simulink model "ScriptDemo"  (R2022b)
settings: configuration reference "TmVcThermal_Configuration_sub" (kept outside this file)
undefined symbols (not defined in the file or in its folder): aaaa, bbbb, cTmComprCtrl_D_u8HvacFlowTable_db, cTmComprCtrl_D_u8HvacFlowTable_sw, cTmComprCtrl_n_i16ChillCmpIMax, cTmComprCtrl_n_i16ChillCmpIMin, cTmComprCtrl_n_i16ChillCmpIMin666, cTmComprCtrl_n_i16ChillCmpPMax, cTmComprCtrl_n_i16ChillCmpPMin, cTmComprCtrl_n_i16CmpChillCoolRpmKiMax, cTmComprCtrl_n_i16CmpChillCoolRpmKiMin, cTmComprCtrl_n_i16CmpChillCoolRpmKpMax, cTmComprCtrl_n_i16CmpChillCoolRpmKpMin, cTmComprCtrl_n_i16CmpCoolRpmKiMax, cTmComprCtrl_n_i16CmpCoolRpmKiMin, cTmComprCtrl_n_i16CmpCoolRpmKpMax, cTmComprCtrl_n_i16CmpCoolRpmKpMin, cTmComprCtrl_n_i16SM4CmpHeatKiMax, cTmComprCtrl_n_i16SM4CmpHeatKiMin, cTmComprCtrl_n_i16SM4CmpHeatKpMax, cTmComprCtrl_n_i16SM4CmpHeatKpMin, cTmComprCtrl_n_i16SM5CmpHeatKiMax, cTmComprCtrl_n_i16SM5CmpHeatKiMin, cTmComprCtrl_n_i16SM5CmpHeatKpMax, cTmComprCtrl_n_i16SM5CmpHeatKpMin, cTmComprCtrl_n_i16SM6CmpHeatKiMax, cTmComprCtrl_n_i16SM6CmpHeatKiMin, cTmComprCtrl_n_i16SM6CmpHeatKpMax, cTmComprCtrl_n_i16SM6CmpHeatKpMin, cTmComprCtrl_n_u16CmpMaxSpdFanFltLimt, cTmComprCtrl_n_u16CmpMaxSpdLoSidePFltLimt, cTmComprCtrl_n_u16CmpMaxSpdSensorFltLimt, cTmComprCtrl_n_u16CompMinRpm, cTmComprCtrl_n_u16CompRpmIncThres, cTmComprCtrl_t_u16BattCooltFFPeriod, cTmComprCtrl_t_u16BattCooltPIPeriod, cTmComprCtrl_t_u16CmpCoolFFPeriod, cTmComprCtrl_t_u16CmpCoolPIPeriod, cTmComprCtrl_t_u16CoolCmpChillFFPeriod, cTmComprCtrl_t_u16CoolCmpChillPIPeriod, cTmComprCtrl_t_u16SM4CmpHeatFFPeriod, cTmComprCtrl_t_u16SM4CmpHeatPIPeriod, cTmComprCtrl_t_u16SM5CmpHeatFFPeriod, cTmComprCtrl_t_u16SM5CmpHeatPIPeriod, cTmComprCtrl_t_u16SM6CmpHeatFFPeriod, cTmComprCtrl_t_u16SM6CmpHeatPIPeriod, cTmComprCtrl_Te_EvapClearInteg, cTmComprCtrl_Te_i16HpReqTempSaturoffset, cTmComprCtrl_Te_i16SatLpReplaceDiff, cTmComprCtrl_Te_i16SM3BatDiffStartEvapDecOffset, cTmComprCtrl_Te_i16SM3EvapLo, cTmComprCtrl_Te_i16SM3TBatDiffEntEvapDecOffset, cTmComprCtrl_Te_i16SM3TBatDiffEntEvapDecOffsetQuit, cTmComprCtrl_Te_s32ErrCmpChillPIContinueCoolH, cTmComprCtrl_Te_s32ErrCmpChillPIContinueCoolL, cTmComprCtrl_Te_s32ErrCmpPIContinueChillH, cTmComprCtrl_Te_s32ErrCmpPIContinueChillL, cTmComprCtrl_Te_s32ErrCmpPIContinueCoolH, cTmComprCtrl_Te_s32ErrCmpPIContinueCoolL, cTmComprCtrl_Te_s32ErrCmpPIContinueHeatH ... (+398)
libraries: simulink x846, PCMULib x711, simulink_need_slupdate x4
(part 33 of 49)

== system ScriptDemo/Create/createMerge/After/SM2SM22/SM2_Kp/Rec ==
  md_u8Blw : Inport
  breakpoint1 : Inport  Port=2
  breakpoint2 : Inport  Port=3
  2-D Lookup Table5 : Lookup_n-D  BreakpointsForDimension1=FFBlw1_Y  BreakpointsForDimension2=FFBlw1_X  BreakpointsForDimension1DataTypeStr=Inherit: Inherit from 'Breakpoint data'  BreakpointsForDimension2DataTypeStr=Inherit: Inherit from 'Breakpoint data'  Table=FFBlw1  TableDataTypeStr=Inherit: Inherit from 'Table data'  ExtrapMethod=Clip  InternalRulePriority=Speed  OutDataTypeStr=Inherit: Inherit from 'Table data'  RndMeth=Simplest
      settings: InputPortMap=u0,u1
  2-D Lookup Table6 : Lookup_n-D  BreakpointsForDimension1=FFBlw3_Y  BreakpointsForDimension2=FFBlw3_X  BreakpointsForDimension1DataTypeStr=Inherit: Inherit from 'Breakpoint data'  BreakpointsForDimension2DataTypeStr=Inherit: Inherit from 'Breakpoint data'  Table=FFBlw3  TableDataTypeStr=Inherit: Inherit from 'Table data'  ExtrapMethod=Clip  InternalRulePriority=Speed  OutDataTypeStr=Inherit: Inherit from 'Table data'  RndMeth=Simplest
      settings: InputPortMap=u0,u1
  2-D Lookup Table7 : Lookup_n-D  BreakpointsForDimension1=FFBlw5_Y  BreakpointsForDimension2=FFBlw5_X  BreakpointsForDimension1DataTypeStr=Inherit: Inherit from 'Breakpoint data'  BreakpointsForDimension2DataTypeStr=Inherit: Inherit from 'Breakpoint data'  Table=FFBlw5  TableDataTypeStr=Inherit: Inherit from 'Table data'  ExtrapMethod=Clip  InternalRulePriority=Speed  OutDataTypeStr=Inherit: Inherit from 'Table data'  RndMeth=Simplest
      settings: InputPortMap=u0,u1
  2-D Lookup Table8 : Lookup_n-D  BreakpointsForDimension1=FFBlw7_Y  BreakpointsForDimension2=FFBlw7_X  BreakpointsForDimension1DataTypeStr=Inherit: Inherit from 'Breakpoint data'  BreakpointsForDimension2DataTypeStr=Inherit: Inherit from 'Breakpoint data'  Table=FFBlw7  TableDataTypeStr=Inherit: Inherit from 'Table data'  ExtrapMethod=Clip  InternalRulePriority=Speed  OutDataTypeStr=Inherit: Inherit from 'Table data'  RndMeth=Simplest
      settings: InputPortMap=u0,u1
  2-D Lookup Table9 : Lookup_n-D  BreakpointsForDimension1=FFBlw9_Y  BreakpointsForDimension2=FFBlw9_X  BreakpointsForDimension1DataTypeStr=Inherit: Inherit from 'Breakpoint data'  BreakpointsForDimension2DataTypeStr=Inherit: Inherit from 'Breakpoint data'  Table=FFBlw9  TableDataTypeStr=Inherit: Inherit from 'Table data'  ExtrapMethod=Clip  InternalRulePriority=Speed  OutDataTypeStr=Inherit: Inherit from 'Table data'  RndMeth=Simplest
      settings: InputPortMap=u0,u1
  Add{2..6} (5 alike) : Sum  Inputs=+-  OutDataTypeStr=int16
  Add7 : Sum  Inputs=+++++
  Constant{,1..4} (5 alike) : Constant  Value=0.1  OutDataTypeStr=single
  Constant5 : Constant  Value=10  OutDataTypeStr=int16
  Constant6 : Constant  Value=20  OutDataTypeStr=int16
  Constant7 : Constant  Value=30  OutDataTypeStr=int16
  Constant8 : Constant  Value=40  OutDataTypeStr=int16
  Constant9 : Constant  Value=50  OutDataTypeStr=int16
  Data Type Conversion : DataTypeConversion  OutDataTypeStr=uint16  SaturateOnIntegerOverflow=off  RndMeth=Floor
  Data Type Conversion1 : DataTypeConversion  OutDataTypeStr=int16  SaturateOnIntegerOverflow=off  RndMeth=Floor
  Product{,1..9} (10 alike) : Product  OutDataTypeStr=single
  Subsystem1 : Subsystem
  Subsystem2 : Subsystem
  Subsystem3 : Subsystem
  Subsystem4 : Subsystem
  Subsystem5 : Subsystem
  XCP : Subsystem
  Flow2Rpm : Outport
  wires:
  Subsystem1/1(Out1) -> Product/2
  Product2/1 -> Product7/2
  [breakpoint2] -> 2-D Lookup Table5/2
  Product4/1 -> Product9/2
  Product9/1 -> Add7/5
  [breakpoint1] -> 2-D Lookup Table7/1
  Constant9/1 -> Add6/1
  [breakpoint1] -> 2-D Lookup Table9/1
  [breakpoint1] -> 2-D Lookup Table5/1
  [breakpoint1] -> 2-D Lookup Table6/1
  Product5/1 -> Add7/1
  2-D Lookup Table7/1 -> Product2/1
  Data Type Conversion1/1 -> Add4/2, Add6/2, Add5/2, Add3/2, Add2/2
  [breakpoint2] -> 2-D Lookup Table8/2
  Product/1 -> Product5/2
  Subsystem5/1(Out1) -> Product4/2
  [breakpoint2] -> 2-D Lookup Table7/2
  Subsystem2/1(Out1) -> Product1/2
  Constant8/1 -> Add5/1
  Product8/1 -> Add7/4
  Constant7/1 -> Add4/1
  Add4/1 -> Subsystem3/1(In1)
  Subsystem3/1(Out1) -> Product2/2
  Subsystem4/1(Out1) -> Product3/2
  Product1/1 -> Product6/2
  Add2/1 -> Subsystem1/1(In1)
  [breakpoint1] -> 2-D Lookup Table8/1
  [breakpoint2] -> 2-D Lookup Table6/2
  2-D Lookup Table5/1 -> Product/1
  Constant5/1 -> Add2/1
  2-D Lookup Table8/1 -> Product3/1
  Constant6/1 -> Add3/1
  Add6/1 -> Subsystem5/1(In1)
  Add5/1 -> Subsystem4/1(In1)
  Product3/1 -> Product8/2
  [breakpoint2] -> 2-D Lookup Table9/2
  Add3/1 -> Subsystem2/1(In1)
  Add7/1 -> Data Type Conversion/1
  2-D Lookup Table6/1 -> Product1/1
  Product7/1 -> Add7/3
  2-D Lookup Table9/1 -> Product4/1
  Product6/1 -> Add7/2
  breakpoint1/1 -> [breakpoint1]
  breakpoint2/1 -> [breakpoint2]
  XCP/1(Out1) -> Data Type Conversion1/1
  Constant/1 -> Product5/1
  Constant1/1 -> Product6/1
  Constant2/1 -> Product7/1
  Constant3/1 -> Product8/1
  Constant4/1 -> Product9/1
  md_u8Blw/1 -> XCP/1(md_u8Blw)
  Data Type Conversion/1 -> Flow2Rpm/1

== system ScriptDemo/Create/createMerge/After/SM3SM23/ID26262_SM3FF/SM1FFEnable ==
  xTmComprCtrl_B_CompOnReqCompOn : Inport  OutDataTypeStr=boolean
  BevvFFPeriod : Subsystem  mask{CounterLim=cTmComprCtrl_t_u16BattCooltFFPeriod}
      mask DialogControl ParameterGroupVar Prompt: 参数
  Compare To Constant2 : simulink/Logic and Bit Operations/Compare To Constant  relop===  const=0  OutDataTypeStr=boolean
  Compare To Constant3 : simulink/Logic and Bit Operations/Compare To Constant  relop===  const=1  OutDataTypeStr=boolean
  Logical Operator3 : Logic  AllPortsSameDT=off  OutDataTypeStr=boolean
  Unit Delay : UnitDelay  SampleTime=-1  HasFrameUpgradeWarning=on
  SM1FFEnable_B_SM1FFEnable : Outport  OutDataTypeStr=boolean
  wires:
  Unit Delay/1 -> Compare To Constant2/1
  [xTmComprCtrl_B_CompOnReqCompOn] -> Compare To Constant3/1, Unit Delay/1
  Compare To Constant2/1 -> Logical Operator3/1
  Logical Operator3/1 -> BevvFFPeriod/1(Counter_Reset)
  BevvFFPeriod/1(Counter_Trig) -> SM1FFEnable_B_SM1FFEnable/1
  Compare To Constant3/1 -> Logical Operator3/2
  xTmComprCtrl_B_CompOnReqCompOn/1 -> [xTmComprCtrl_B_CompOnReqCompOn]

== system ScriptDemo/Create/createMerge/After/SM3SM23/ID26262_SM3FF/SM2FFEnable ==
  xTmComprCtrl_B_CompOnReqCompOn : Inport  OutDataTypeStr=boolean
  Compare To Constant2 : simulink/Logic and Bit Operations/Compare To Constant  relop===  const=0  OutDataTypeStr=boolean
  Compare To Constant3 : simulink/Logic and Bit Operations/Compare To Constant  relop===  const=1  OutDataTypeStr=boolean
  Logical Operator3 : Logic  AllPortsSameDT=off  OutDataTypeStr=boolean
  PeriodTrig : Subsystem  mask{CounterLim=cTmComprCtrl_t_u16CoolCmpChillFFPeriod}
      mask DialogControl ParameterGroupVar Prompt: 参数
  Unit Delay : UnitDelay  SampleTime=-1  HasFrameUpgradeWarning=on
  SM2FFEnable_B_SM2FFEnable : Outport  OutDataTypeStr=boolean
  wires:
  Unit Delay/1 -> Compare To Constant2/1
  [xTmComprCtrl_B_CompOnReqCompOn] -> Compare To Constant3/1, Unit Delay/1
  Compare To Constant2/1 -> Logical Operator3/1
  Logical Operator3/1 -> PeriodTrig/1(Counter_Reset)
  Compare To Constant3/1 -> Logical Operator3/2
  xTmComprCtrl_B_CompOnReqCompOn/1 -> [xTmComprCtrl_B_CompOnReqCompOn]
  PeriodTrig/1(Counter_Trig) -> SM2FFEnable_B_SM2FFEnable/1

== system ScriptDemo/Create/createMerge/After/SM3SM23/ID26262_SM3FF/SM3SM1FF ==
  sTmIn_D_u8DCChrgSt : Inport  OutDataTypeStr=uint8
  sTmSigProces_D_u8HvBattCoolgReq : Inport  Port=2  OutDataTypeStr=uint8
  sTmIn_D_u8HeatPump : Inport  Port=3  OutDataTypeStr=uint8
  Enable : EnablePort
  1-D Lookup Table1 : Lookup_n-D  NumberOfTableDimensions=1  BreakpointsForDimension1=tTmComprCtrl_fac_s32SM1FFTFactor_X  BreakpointsForDimension1DataTypeStr=Inherit: Inherit from 'Breakpoint data'  Table=tTmComprCtrl_fac_s32SM1FFTFactor  TableDataTypeStr=Inherit: Inherit from 'Table data'  ExtrapMethod=Clip  InternalRulePriority=Speed  OutDataTypeStr=Inherit: Inherit via back propagation  RndMeth=Simplest  InputSameDT=off
  2-D Lookup Table1 : Lookup_n-D  BreakpointsForDimension1=mTmComprCtrl_n_u16FFBattCooltRpmNorm_Y  BreakpointsForDimension2=mTmComprCtrl_n_u16FFBattCooltRpmNorm_X  BreakpointsForDimension1DataTypeStr=Inherit: Inherit from 'Breakpoint data'  BreakpointsForDimension2DataTypeStr=Inherit: Inherit from 'Breakpoint data'  Table=mTmComprCtrl_n_u16FFBattCooltRpmNorm  TableDataTypeStr=Inherit: Inherit from 'Table data'  ExtrapMethod=Clip  InternalRulePriority=Speed  OutDataTypeStr=Inherit: Inherit via back propagation  RndMeth=Simplest  InputSameDT=off
      settings: InputPortMap=u0,u1
  2-D Lookup Table2 : Lookup_n-D  BreakpointsForDimension1=mTmComprCtrl_n_u16FFBattCooltRpmNormNhp_Y  BreakpointsForDimension2=mTmComprCtrl_n_u16FFBattCooltRpmNormNhp_X  BreakpointsForDimension1DataTypeStr=Inherit: Inherit from 'Breakpoint data'  BreakpointsForDimension2DataTypeStr=Inherit: Inherit from 'Breakpoint data'  Table=mTmComprCtrl_n_u16FFBattCooltRpmNormNhp  TableDataTypeStr=Inherit: Inherit from 'Table data'  ExtrapMethod=Clip  InternalRulePriority=Speed  OutDataTypeStr=Inherit: Inherit via back propagation  RndMeth=Simplest  InputSameDT=off
      settings: InputPortMap=u0,u1
  2-D Lookup Table5 : Lookup_n-D  LookupTableObject=mTmComprCtrl_n_u16FFBattCooltRpmCharging  BreakpointsForDimension1=mTmComprCtrl_n_u16FFBattCooltRpmChargingNhp_Y  BreakpointsForDimension2=mTmComprCtrl_n_u16FFBattCooltRpmChargingNhp_X  BreakpointsForDimension1DataTypeStr=Inherit: Inherit from 'Breakpoint data'  BreakpointsForDimension2DataTypeStr=Inherit: Inherit from 'Breakpoint data'  Table=mTmComprCtrl_n_u16FFBattCooltRpmChargingNhp  TableDataTypeStr=Inherit: Inherit from 'Table data'  ExtrapMethod=Clip  InternalRulePriority=Speed  OutDataTypeStr=Inherit: Inherit via back propagation  RndMeth=Simplest  InputSameDT=off
      settings: InputPortMap=u0,u1
  2-D Lookup Table6 : Lookup_n-D  LookupTableObject=mTmComprCtrl_n_u16FFBattCooltRpmCharging  BreakpointsForDimension1=mTmComprCtrl_n_u16FFBattCooltRpmCharging_Y  BreakpointsForDimension2=mTmComprCtrl_n_u16FFBattCooltRpmCharging_X  BreakpointsForDimension1DataTypeStr=Inherit: Inherit from 'Breakpoint data'  BreakpointsForDimension2DataTypeStr=Inherit: Inherit from 'Breakpoint data'  Table=mTmComprCtrl_n_u16FFBattCooltRpmCharging  TableDataTypeStr=Inherit: Inherit from 'Table data'  ExtrapMethod=Clip  InternalRulePriority=Speed  OutDataTypeStr=Inherit: Inherit via back propagation  RndMeth=Simplest  InputSameDT=off
      settings: InputPortMap=u0,u1
  2-D Lookup Table7 : Lookup_n-D  LookupTableObject=mTmComprCtrl_n_u16FFBattCooltRpmCharging  BreakpointsForDimension1=mTmComprCtrl_n_u16FFBattCooltRpmSuperCharging_Y  BreakpointsForDimension2=mTmComprCtrl_n_u16FFBattCooltRpmSuperCharging_X  BreakpointsForDimension1DataTypeStr=Inherit: Inherit from 'Breakpoint data'  BreakpointsForDimension2DataTypeStr=Inherit: Inherit from 'Breakpoint data'  Table=mTmComprCtrl_n_u16FFBattCooltRpmSuperCharging  TableDataTypeStr=Inherit: Inherit from 'Table data'  ExtrapMethod=Clip  InternalRulePriority=Speed  OutDataTypeStr=Inherit: Inherit via back propagation  RndMeth=Simplest  InputSameDT=off
      settings: InputPortMap=u0,u1
  2-D Lookup Table8 : Lookup_n-D  LookupTableObject=mTmComprCtrl_n_u16FFBattCooltRpmCharging  BreakpointsForDimension1=mTmComprCtrl_n_u16FFBattCooltRpmSuperChargingNhp_Y  BreakpointsForDimension2=mTmComprCtrl_n_u16FFBattCooltRpmSuperChargingNhp_X  BreakpointsForDimension1DataTypeStr=Inherit: Inherit from 'Breakpoint data'  BreakpointsForDimension2DataTypeStr=Inherit: Inherit from 'Breakpoint data'  Table=mTmComprCtrl_n_u16FFBattCooltRpmSuperChargingNhp  TableDataTypeStr=Inherit: Inherit from 'Table data'  ExtrapMethod=Clip  InternalRulePriority=Speed  OutDataTypeStr=Inherit: Inherit via back propagation  RndMeth=Simplest  InputSameDT=off
      settings: InputPortMap=u0,u1
  Compare To Constant : simulink/Logic and Bit Operations/Compare To Constant  relop===  const=2  OutDataTypeStr=boolean
  Multiport Switch : MultiPortSwitch  DataPortOrder=Specify indices  DataPortIndices={2,12}  DataPortForDefault=Additional data port  DiagnosticForDefault=None  SaturateOnIntegerOverflow=off  InputSameDT=off
  Multiport Switch1 : MultiPortSwitch  DataPortOrder=Specify indices  DataPortIndices={2,12}  DataPortForDefault=Additional data port  DiagnosticForDefault=None  SaturateOnIntegerOverflow=off  InputSameDT=off
  Product1 : Product  OutDataTypeStr=uint16
  Switch : Switch  Criteria=u2 ~= 0  SaturateOnIntegerOverflow=off  InputSameDT=off
  SM1FF : Outport
  wires:
  ? -> [sTmIn_Te_s32HvBattCooltTReq]
  sTmIn_D_u8DCChrgSt/1 -> [sTmIn_D_u8DCChrgSt]
  sTmSigProces_D_u8HvBattCoolgReq/1 -> [sTmSigProces_D_u8HvBattCoolgReq]
  ? -> [sTmSigProces_Te_s32TAmb]
  Multiport Switch1/1 -> Switch/3
  Switch/1 -> Product1/1  "rTmComprCtrl_fac_s32SM3SM1FFRaw"
  2-D Lookup Table5/1 -> Multiport Switch1/3
  [sTmSigProces_D_u8HvBattCoolgReq] -> 2-D Lookup Table8/1, 2-D Lookup Table5/1, 2-D Lookup Table2/1
  [sTmIn_D_u8DCChrgSt] -> Multiport Switch1/1
  2-D Lookup Table8/1 -> Multiport Switch1/4
  2-D Lookup Table2/1 -> Multiport Switch1/2
  2-D Lookup Table1/1 -> Multiport Switch/2
  Compare To Constant/1 -> Switch/2
  [sTmIn_D_u8DCChrgSt] -> Multiport Switch/1
  2-D Lookup Table6/1 -> Multiport Switch/3
  [sTmIn_D_u8HeatPump] -> Compare To Constant/1
  2-D Lookup Table7/1 -> Multiport Switch/4
  Multiport Switch/1 -> Switch/1
  [sTmSigProces_Te_s32TAmb] -> 1-D Lookup Table1/1
  Product1/1 -> SM1FF/1  "SM1FF"
  [sTmSigProces_D_u8HvBattCoolgReq] -> 2-D Lookup Table7/1, 2-D Lookup Table6/1, 2-D Lookup Table1/1
  1-D Lookup Table1/1 -> Product1/2  "rTmComprCtrl_fac_s32SM3SM1FFTFactor"
  [sTmIn_Te_s32HvBattCooltTReq] -> 2-D Lookup Table7/2, 2-D Lookup Table6/2, 2-D Lookup Table1/2
  [sTmIn_Te_s32HvBattCooltTReq] -> 2-D Lookup Table8/2, 2-D Lookup Table5/2, 2-D Lookup Table2/2
  sTmIn_D_u8HeatPump/1 -> [sTmIn_D_u8HeatPump]

== system ScriptDemo/Create/createMerge/After/SM3SM23/ID26262_SM3FF/SM3SM2FF ==
  note: FF
  sTmSigProces_Te_s32EvapFanReqRamp : Inport  OutDataTypeStr=single
  sTmIn_X_s32ClimtRcirc : Inport  Port=2  OutDataTypeStr=single
  sTmComprCtrl_D_u8HvacFlowLevel : Inport  Port=3  OutDataTypeStr=uint8
  sTmIn_D_u8HeatPump : Inport  Port=4  OutDataTypeStr=uint8
  Enable : EnablePort
  Compare To Constant : simulink/Logic and Bit Operations/Compare To Constant  relop===  const=2  OutDataTypeStr=boolean
  Demux : Demux  Outputs=2
  Flow2RpmOsa : Subsystem  mask{BlwHeatLevel_db=cTmComprCtrl_D_u8HvacFlowTable_db, BlwHeatLevel_sw=cTmComprCtrl_D_u8HvacFlowTable_sw, FFBlw1=mTmComprCtrl_n_u16FFCmpCoolRpm_OsaFlow1, FFBlw1_Y=mTmComprCtrl_n_u16FFCmpCoolRpm_OsaFlow1_Y, FFBlw1_X=mTmComprCtrl_n_u16FFCmpCoolRpm_OsaFlow1_X, FFBlw3=mTmComprCtrl_n_u16FFCmpCoolRpm_OsaFlow3, FFBlw3_Y=mTmComprCtrl_n_u16FFCmpCoolRpm_OsaFlow3_Y, FFBlw3_X=mTmComprCtrl_n_u16FFCmpCoolRpm_OsaFlow3_X, FFBlw5=mTmComprCtrl_n_u16FFCmpCoolRpm_OsaFlow5, FFBlw5_Y=mTmComprCtrl_n_u16FFCmpCoolRpm_OsaFlow5_Y, FFBlw5_X=mTmComprCtrl_n_u16FFCmpCoolRpm_OsaFlow5_X, FFBlw7=mTmComprCtrl_n_u16FFCmpCoolRpm_OsaFlow7, FFBlw7_Y=mTmComprCtrl_n_u16FFCmpCoolRpm_OsaFlow7_Y, FFBlw7_X=mTmComprCtrl_n_u16FFCmpCoolRpm_OsaFlow7_X, FFBlw9=mTmComprCtrl_n_u16FFCmpCoolRpm_OsaFlow9, FFBlw9_Y=mTmComprCtrl_n_u16FFCmpCoolRpm_OsaFlow9_Y, FFBlw9_X=mTmComprCtrl_n_u16FFCmpCoolRpm_OsaFlow9_X}
      mask DialogControl ParameterGroupVar Prompt: 参数
  Flow2RpmOsa1 : Subsystem  mask{BlwHeatLevel_db=cTmComprCtrl_D_u8HvacFlowTable_db, BlwHeatLevel_sw=cTmComprCtrl_D_u8HvacFlowTable_sw, FFBlw1=mTmComprCtrl_n_u16FFCmpCoolRpmNhpOsaFlow1, FFBlw1_Y=mTmComprCtrl_n_u16FFCmpCoolRpmNhpOsaFlow1_Y, FFBlw1_X=mTmComprCtrl_n_u16FFCmpCoolRpmNhpOsaFlow1_X, FFBlw3=mTmComprCtrl_n_u16FFCmpCoolRpmNhpOsaFlow3, FFBlw3_Y=mTmComprCtrl_n_u16FFCmpCoolRpmNhpOsaFlow3_Y, FFBlw3_X=mTmComprCtrl_n_u16FFCmpCoolRpmNhpOsaFlow3_X, FFBlw5=mTmComprCtrl_n_u16FFCmpCoolRpmNhpOsaFlow5, FFBlw5_Y=mTmComprCtrl_n_u16FFCmpCoolRpmNhpOsaFlow5_Y, FFBlw5_X=mTmComprCtrl_n_u16FFCmpCoolRpmNhpOsaFlow5_X, FFBlw7=mTmComprCtrl_n_u16FFCmpCoolRpmNhpOsaFlow7, FFBlw7_Y=mTmComprCtrl_n_u16FFCmpCoolRpmNhpOsaFlow7_Y, FFBlw7_X=mTmComprCtrl_n_u16FFCmpCoolRpmNhpOsaFlow7_X, FFBlw9=mTmComprCtrl_n_u16FFCmpCoolRpmNhpOsaFlow9, FFBlw9_Y=mTmComprCtrl_n_u16FFCmpCoolRpmNhpOsaFlow9_Y, FFBlw9_X=mTmComprCtrl_n_u16FFCmpCoolRpmNhpOsaFlow9_X}
      mask DialogControl ParameterGroupVar Prompt: 参数
  Flow2RpmRec : Subsystem  mask{BlwHeatLevel_db=cTmComprCtrl_D_u8HvacFlowTable_db, BlwHeatLevel_sw=cTmComprCtrl_D_u8HvacFlowTable_sw, FFBlw1=mTmComprCtrl_n_u16FFCmpCoolRpm_RecFlow1, FFBlw1_Y=mTmComprCtrl_n_u16FFCmpCoolRpm_RecFlow1_Y, FFBlw1_X=mTmComprCtrl_n_u16FFCmpCoolRpm_RecFlow1_X, FFBlw3=mTmComprCtrl_n_u16FFCmpCoolRpm_RecFlow3, FFBlw3_Y=mTmComprCtrl_n_u16FFCmpCoolRpm_RecFlow3_Y, FFBlw3_X=mTmComprCtrl_n_u16FFCmpCoolRpm_RecFlow3_X, FFBlw5=mTmComprCtrl_n_u16FFCmpCoolRpm_RecFlow5, FFBlw5_Y=mTmComprCtrl_n_u16FFCmpCoolRpm_RecFlow5_Y, FFBlw5_X=mTmComprCtrl_n_u16FFCmpCoolRpm_RecFlow5_X, FFBlw7=mTmComprCtrl_n_u16FFCmpCoolRpm_RecFlow7, FFBlw7_Y=mTmComprCtrl_n_u16FFCmpCoolRpm_RecFlow7_Y, FFBlw7_X=mTmComprCtrl_n_u16FFCmpCoolRpm_RecFlow7_X, FFBlw9=mTmComprCtrl_n_u16FFCmpCoolRpm_RecFlow9, FFBlw9_Y=mTmComprCtrl_n_u16FFCmpCoolRpm_RecFlow9_Y, FFBlw9_X=mTmComprCtrl_n_u16FFCmpCoolRpm_RecFlow9_X}
      mask DialogControl ParameterGroupVar Prompt: 参数
  Flow2RpmRec1 : Subsystem  mask{BlwHeatLevel_db=cTmComprCtrl_D_u8HvacFlowTable_db, BlwHeatLevel_sw=cTmComprCtrl_D_u8HvacFlowTable_sw, FFBlw1=mTmComprCtrl_n_u16FFCmpCoolRpmNhpRecFlow1, FFBlw1_Y=mTmComprCtrl_n_u16FFCmpCoolRpmNhpRecFlow1_Y, FFBlw1_X=mTmComprCtrl_n_u16FFCmpCoolRpmNhpRecFlow1_X, FFBlw3=mTmComprCtrl_n_u16FFCmpCoolRpmNhpRecFlow3, FFBlw3_Y=mTmComprCtrl_n_u16FFCmpCoolRpmNhpRecFlow3_Y, FFBlw3_X=mTmComprCtrl_n_u16FFCmpCoolRpmNhpRecFlow3_X, FFBlw5=mTmComprCtrl_n_u16FFCmpCoolRpmNhpRecFlow5, FFBlw5_Y=mTmComprCtrl_n_u16FFCmpCoolRpmNhpRecFlow5_Y, FFBlw5_X=mTmComprCtrl_n_u16FFCmpCoolRpmNhpRecFlow5_X, FFBlw7=mTmComprCtrl_n_u16FFCmpCoolRpmNhpRecFlow7, FFBlw7_Y=mTmComprCtrl_n_u16FFCmpCoolRpmNhpRecFlow7_Y, FFBlw7_X=mTmComprCtrl_n_u16FFCmpCoolRpmNhpRecFlow7_X, FFBlw9=mTmComprCtrl_n_u16FFCmpCoolRpmNhpRecFlow9, FFBlw9_Y=mTmComprCtrl_n_u16FFCmpCoolRpmNhpRecFlow9_Y, FFBlw9_X=mTmComprCtrl_n_u16FFCmpCoolRpmNhpRecFlow9_X}
      mask DialogControl ParameterGroupVar Prompt: 参数
  Mux : Mux  Inputs=2
  Mux1 : Mux  Inputs=2
  Signal Conversion : SignalConversion  OverrideOpt=off
  Signal Conversion1 : SignalConversion  OverrideOpt=off
  Switch : Switch  Criteria=u2 ~= 0  SaturateOnIntegerOverflow=off  InputSameDT=off
  interpolation : PCMULib/Calculation/interpolation  SystemSampleTime=-1  VariantActivationTime=update diagram  Latency=0  AutoFrameSizeCalculation=off
      settings: SourceProductName=PCMULib
  SM2FF : Outport  OutDataTypeStr=uint16
  wires:
  [sTmIn_X_s32ClimtRcirc] -> interpolation/1
  interpolation/1 -> SM2FF/1
  sTmSigProces_Te_s32EvapFanReqRamp/1 -> [sTmSigProces_Te_s32EvapFanReqRamp]
  ? -> [sTmSigProces_Te_s32TAmb]
  sTmIn_X_s32ClimtRcirc/1 -> [sTmIn_X_s32ClimtRcirc]
  sTmComprCtrl_D_u8HvacFlowLevel/1 -> [sTmComprCtrl_D_u8HvacFlowLevel]
  [sTmComprCtrl_D_u8HvacFlowLevel] -> Flow2RpmRec/1(md_u8Blw)
  [sTmSigProces_Te_s32TAmb] -> Flow2RpmRec/2(breakpoint1)
  [sTmSigProces_Te_s32EvapFanReqRamp] -> Flow2RpmRec/3(breakpoint2)
  [sTmComprCtrl_D_u8HvacFlowLevel] -> Flow2RpmOsa/1(md_u8Blw)
  [sTmSigProces_Te_s32EvapFanReqRamp] -> Flow2RpmOsa/3(breakpoint2)
  [sTmSigProces_Te_s32TAmb] -> Flow2RpmOsa/2(breakpoint1)
  [sTmIn_D_u8HeatPump] -> Compare To Constant/1
  Compare To Constant/1 -> Switch/2
  Flow2RpmOsa/1(Flow2Rpm) -> Mux/2
  Flow2RpmRec/1(Flow2Rpm) -> Mux/1
  Mux/1 -> Switch/1
  [sTmSigProces_Te_s32TAmb] -> Flow2RpmOsa1/2(breakpoint1)
  [sTmSigProces_Te_s32TAmb] -> Flow2RpmRec1/2(breakpoint1)
  [sTmSigProces_Te_s32EvapFanReqRamp] -> Flow2RpmRec1/3(breakpoint2)
  [sTmComprCtrl_D_u8HvacFlowLevel] -> Flow2RpmRec1/1(md_u8Blw)
  [sTmSigProces_Te_s32EvapFanReqRamp] -> Flow2RpmOsa1/3(breakpoint2)
  [sTmComprCtrl_D_u8HvacFlowLevel] -> Flow2RpmOsa1/1(md_u8Blw)
  Flow2RpmRec1/1(Flow2Rpm) -> Mux1/1
  Flow2RpmOsa1/1(Flow2Rpm) -> Mux1/2
  Mux1/1 -> Switch/3
  Demux/2 -> Signal Conversion1/1
  Demux/1 -> Signal Conversion/1
  sTmIn_D_u8HeatPump/1 -> [sTmIn_D_u8HeatPump]
  Signal Conversion/1 -> interpolation/2  "rTmComprCtrl_n_u16ComprRpmFFSM3Rec"
  Signal Conversion1/1 -> interpolation/3  "rTmComprCtrl_n_u16ComprRpmFFSM3Osa"
  Switch/1 -> Demux/1

== system ScriptDemo/Create/createMerge/After/SM3SM23/ID26263_SM3Error/SM3HPErr ==
  sTmSigProces_Te_s32EvapFanReqRamp : Inport  OutDataTypeStr=single
  sTmSigProces_Te_s32EvapFanFilter : Inport  Port=2  OutDataTypeStr=single
  xTmComprCtrl_B_ModeChanged : Inport  Port=3  OutDataTypeStr=boolean
  Add5 : Sum  Inputs=-+
  CalEvapReqOffset : Subsystem
  NegAndPosCheck 1 : Subsystem  AncestorBlock=CustomLib/TempNegAndPosCheck
  Terminator : Terminator
  isNeedOffset : Subsystem
  SM3HPErr_Te_s32Error : Outport
  wires:
  [sTmSigProces_Te_s32EvapFanFilter] -> NegAndPosCheck 1/2(Acture)
  [sTmSigProces_Te_s32EvapFanReqRamp] -> Add5/2
  NegAndPosCheck 1/2(Dvt_PosFlag) -> Terminator/1
  [rTmComprCtrl_Te_s32SM3EvapReqOffset] -> Add5/1
  Add5/1 -> NegAndPosCheck 1/1(SetPoint)
  NegAndPosCheck 1/1(Dvt) -> SM3HPErr_Te_s32Error/1
  CalEvapReqOffset/1(rTmComprCtrl_Te_s32SM3EvapReqOffset) -> [rTmComprCtrl_Te_s32SM3EvapReqOffset]
  sTmSigProces_Te_s32EvapFanReqRamp/1 -> [sTmSigProces_Te_s32EvapFanReqRamp]
  ? -> [sTmIn_Te_s32HvBattCooltTReq]
  sTmSigProces_Te_s32EvapFanFilter/1 -> [sTmSigProces_Te_s32EvapFanFilter]
  ? -> [sTmSigProces_Te_s32HvBattCooltTFilter]
  xTmComprCtrl_B_ModeChanged/1 -> [xTmComprCtrl_B_ModeChanged]
  [sTmSigProces_Te_s32EvapFanFilter] -> isNeedOffset/1(sTmSigProces_Te_s32EvapFanFilter)
  [sTmIn_Te_s32HvBattCooltTReq] -> ?
  [sTmSigProces_Te_s32HvBattCooltTFilter] -> ?
  isNeedOffset/1(xTmComprCtrl_B_SM3ErrNeedOffset) -> [xTmComprCtrl_B_SM3ErrNeedOffset]
  isNeedOffset/2(rTmComprCtrl_Te_s32SM3BattError) -> [rTmComprCtrl_Te_s32SM3BattError]
  [sTmSigProces_Te_s32EvapFanReqRamp] -> CalEvapReqOffset/1(sTmSigProces_Te_s32EvapFanReqRamp)
  [xTmComprCtrl_B_ModeChanged] -> CalEvapReqOffset/2(xTmComprCtrl_B_ModeChanged)
  [rTmComprCtrl_Te_s32SM3BattError] -> CalEvapReqOffset/3(rTmComprCtrl_Te_s32SM3BattError)
  [xTmComprCtrl_B_SM3ErrNeedOffset] -> CalEvapReqOffset/4(xTmComprCtrl_B_SM3ErrNeedOffset)

== system ScriptDemo/Create/createMerge/After/SM3SM23/ID26263_SM3Error/SM3NHPErr ==
  sTmSigProces_Te_s32EvapFanReqRamp : Inport  OutDataTypeStr=single
  sTmSigProces_D_u8HvBattCoolgReq : Inport  Port=2  OutDataTypeStr=uint8
  sTmSigProces_Te_s32EvapFanFilter : Inport  Port=3  OutDataTypeStr=single
  Compare To Constant2 : simulink/Logic and Bit Operations/Compare To Constant  relop===  const=3  OutDataTypeStr=boolean
  NegAndPosCheck 2 : Subsystem  AncestorBlock=CustomLib/TempNegAndPosCheck
  NegAndPosCheck 3 : Subsystem  AncestorBlock=CustomLib/TempNegAndPosCheck
  Switch5 : Switch  Criteria=u2 ~= 0  SaturateOnIntegerOverflow=off  InputSameDT=off
  Terminator1 : Terminator
  Terminator2 : Terminator
  SM3NHPErr_Te_s32Error : Outport  OutDataTypeStr=single
  wires:
  NegAndPosCheck 2/2(Dvt_PosFlag) -> Terminator1/1
  NegAndPosCheck 2/1(Dvt) -> Switch5/1
  NegAndPosCheck 3/2(Dvt_PosFlag) -> Terminator2/1
  [sTmSigProces_Te_s32EvapFanFilter] -> NegAndPosCheck 3/2(Acture)
  [sTmSigProces_Te_s32EvapFanReqRamp] -> NegAndPosCheck 3/1(SetPoint)
  Compare To Constant2/1 -> Switch5/2
  NegAndPosCheck 3/1(Dvt) -> Switch5/3
  Switch5/1 -> [SM3NHPErr_Te_s32Error]
  [sTmSigProces_Te_s32HvBattCooltTFilter] -> NegAndPosCheck 2/2(Acture)
  [sTmIn_Te_s32HvBattCooltTReq] -> NegAndPosCheck 2/1(SetPoint)
  [sTmSigProces_D_u8HvBattCoolgReq] -> Compare To Constant2/1
  sTmSigProces_Te_s32EvapFanReqRamp/1 -> [sTmSigProces_Te_s32EvapFanReqRamp]
  ? -> [sTmIn_Te_s32HvBattCooltTReq]
  sTmSigProces_D_u8HvBattCoolgReq/1 -> [sTmSigProces_D_u8HvBattCoolgReq]
  sTmSigProces_Te_s32EvapFanFilter/1 -> [sTmSigProces_Te_s32EvapFanFilter]
  ? -> [sTmSigProces_Te_s32HvBattCooltTFilter]
  [SM3NHPErr_Te_s32Error] -> SM3NHPErr_Te_s32Error/1

== system ScriptDemo/Create/createMerge/After/SM3SM23/SM3SM1Error/NegAndPosCheck  ==
  SetPoint : Inport
  Acture : Inport  Port=2
  Compare To Constant : simulink/Logic and Bit Operations/Compare To Constant  relop=>=  const=0  OutDataTypeStr=boolean
  Data Type Conversion : DataTypeConversion  SaturateOnIntegerOverflow=off  RndMeth=Floor
  Data Type Conversion1 : DataTypeConversion  SaturateOnIntegerOverflow=off  RndMeth=Floor
  Data Type Conversion2 : DataTypeConversion  SaturateOnIntegerOverflow=off  RndMeth=Floor
  Sum : Sum  Inputs=|-+  OutDataTypeStr=Inherit: Same as first input
  Dvt : Outport  VectorParamsAs1DForOutWhenUnconnected=off
  Dvt_PosFlag : Outport  Port=2  VectorParamsAs1DForOutWhenUnconnected=off
  wires:
  SetPoint/1 -> Data Type Conversion/1
  Acture/1 -> Data Type Conversion1/1
  Sum/1 -> Data Type Conversion2/1
  Compare To Constant/1 -> Dvt_PosFlag/1
  Data Type Conversion/1 -> Sum/1
  Data Type Conversion1/1 -> Sum/2
  Data Type Conversion2/1 -> Compare To Constant/1, Dvt/1

== system ScriptDemo/Create/createMerge/After/SM3SM23/SM3SM2Error/NegAndPosCheck 1 ==
  SetPoint : Inport
  Acture : Inport  Port=2
  Compare To Constant : simulink/Logic and Bit Operations/Compare To Constant  relop=>=  const=0  OutDataTypeStr=boolean
  Data Type Conversion : DataTypeConversion  SaturateOnIntegerOverflow=off  RndMeth=Floor
  Data Type Conversion1 : DataTypeConversion  SaturateOnIntegerOverflow=off  RndMeth=Floor
  Data Type Conversion2 : DataTypeConversion  SaturateOnIntegerOverflow=off  RndMeth=Floor
  Sum : Sum  Inputs=|-+  OutDataTypeStr=Inherit: Same as first input
  Dvt : Outport  VectorParamsAs1DForOutWhenUnconnected=off
  Dvt_PosFlag : Outport  Port=2  VectorParamsAs1DForOutWhenUnconnected=off
  wires:
  Data Type Conversion2/1 -> Dvt/1, Compare To Constant/1
  Data Type Conversion1/1 -> Sum/2
  Data Type Conversion/1 -> Sum/1
  Compare To Constant/1 -> Dvt_PosFlag/1
  Sum/1 -> Data Type Conversion2/1
  Acture/1 -> Data Type Conversion1/1
  SetPoint/1 -> Data Type Conversion/1

== system ScriptDemo/Create/createMerge/After/SM3SM23/SM3_Ki/SM1Ki ==
  sTmSigProces_D_u8BattThermReq : Inport
  sTmIn_D_u8DCChrgSt : Inport  Port=2
  sTmSigProces_D_u8HvBattCoolgReq : Inport  Port=3
  Error : Inport  Port=4
  2-D Lookup Table10 : Lookup_n-D  LookupTableObject=mTmComprCtrl_n_u16FFBattCooltRpmCharging  BreakpointsForDimension1=mTmComprCtrl_n_u16KiBattCooltRpmSuperCharging_Y  BreakpointsForDimension2=mTmComprCtrl_n_u16KiBattCooltRpmSuperCharging_X  BreakpointsForDimension1DataTypeStr=Inherit: Inherit from 'Breakpoint data'  BreakpointsForDimension2DataTypeStr=Inherit: Inherit from 'Breakpoint data'  Table=mTmComprCtrl_n_u16KiBattCooltRpmSuperCharging  TableDataTypeStr=Inherit: Inherit from 'Table data'  ExtrapMethod=Clip  InternalRulePriority=Speed  OutDataTypeStr=Inherit: Inherit via back propagation  RndMeth=Simplest  InputSameDT=off
      settings: InputPortMap=u0,u1
  2-D Lookup Table8 : Lookup_n-D  LookupTableObject=mTmComprCtrl_n_u16FFBattCooltRpmCharging  BreakpointsForDimension1=mTmComprCtrl_n_u16KiBattCooltRpmNorm_Y  BreakpointsForDimension2=mTmComprCtrl_n_u16KiBattCooltRpmNorm_X  BreakpointsForDimension1DataTypeStr=Inherit: Inherit from 'Breakpoint data'  BreakpointsForDimension2DataTypeStr=Inherit: Inherit from 'Breakpoint data'  Table=mTmComprCtrl_n_u16KiBattCooltRpmNorm  TableDataTypeStr=Inherit: Inherit from 'Table data'  ExtrapMethod=Clip  InternalRulePriority=Speed  OutDataTypeStr=Inherit: Inherit via back propagation  RndMeth=Simplest  InputSameDT=off
      settings: InputPortMap=u0,u1
  2-D Lookup Table9 : Lookup_n-D  LookupTableObject=mTmComprCtrl_n_u16FFBattCooltRpmCharging  BreakpointsForDimension1=mTmComprCtrl_n_u16KiBattCooltRpmCharging_Y  BreakpointsForDimension2=mTmComprCtrl_n_u16KiBattCooltRpmCharging_X  BreakpointsForDimension1DataTypeStr=Inherit: Inherit from 'Breakpoint data'  BreakpointsForDimension2DataTypeStr=Inherit: Inherit from 'Breakpoint data'  Table=mTmComprCtrl_n_u16KiBattCooltRpmCharging  TableDataTypeStr=Inherit: Inherit from 'Table data'  ExtrapMethod=Clip  InternalRulePriority=Speed  OutDataTypeStr=Inherit: Inherit via back propagation  RndMeth=Simplest  InputSameDT=off
      settings: InputPortMap=u0,u1
  tableChoose : Subsystem
  SM1Ki : Outport
  wires:
  sTmIn_D_u8DCChrgSt/1 -> tableChoose/2(sTmIn_D_u8DCChrgSt)
  sTmSigProces_D_u8BattThermReq/1 -> tableChoose/1(sTmSigProces_D_u8BattThermReq)
  2-D Lookup Table10/1 -> tableChoose/5(tab3)
  2-D Lookup Table8/1 -> tableChoose/3(tab1)
  2-D Lookup Table9/1 -> tableChoose/4(tab2)
  tableChoose/1(out) -> SM1Ki/1
  sTmSigProces_D_u8HvBattCoolgReq/1 -> 2-D Lookup Table8/1, 2-D Lookup Table10/1, 2-D Lookup Table9/1
  Error/1 -> 2-D Lookup Table8/2, 2-D Lookup Table10/2, 2-D Lookup Table9/2

== system ScriptDemo/Create/createMerge/After/SM3SM23/SM3_Ki/SM2Ki ==
  Error : Inport
  sTmIn_X_s32ClimtRcirc : Inport  Port=2  OutDataTypeStr=single
  sTmComprCtrl_D_u8HvacFlowLevel : Inport  Port=3  OutDataTypeStr=uint8
  Flow2Rpm : Subsystem  mask{BlwHeatLevel_db=cTmComprCtrl_D_u8HvacFlowTable_db, BlwHeatLevel_sw=cTmComprCtrl_D_u8HvacFlowTable_sw, FFBlw1=mTmComprCtrl_n_u16KiCmpCoolRpm_RecFlow1, FFBlw1_Y=mTmComprCtrl_n_u16KiCmpCoolRpm_RecFlow1_Y, FFBlw1_X=mTmComprCtrl_n_u16KiCmpCoolRpm_RecFlow1_X, FFBlw3=mTmComprCtrl_n_u16KiCmpCoolRpm_RecFlow3, FFBlw3_Y=mTmComprCtrl_n_u16KiCmpCoolRpm_RecFlow3_Y, FFBlw3_X=mTmComprCtrl_n_u16KiCmpCoolRpm_RecFlow3_X, FFBlw5=mTmComprCtrl_n_u16KiCmpCoolRpm_RecFlow5, FFBlw5_Y=mTmComprCtrl_n_u16KiCmpCoolRpm_RecFlow5_Y, FFBlw5_X=mTmComprCtrl_n_u16KiCmpCoolRpm_RecFlow5_X, FFBlw7=mTmComprCtrl_n_u16KiCmpCoolRpm_RecFlow7, FFBlw7_Y=mTmComprCtrl_n_u16KiCmpCoolRpm_RecFlow7_Y, FFBlw7_X=mTmComprCtrl_n_u16KiCmpCoolRpm_RecFlow7_X, FFBlw9=mTmComprCtrl_n_u16KiCmpCoolRpm_RecFlow9, FFBlw9_Y=mTmComprCtrl_n_u16KiCmpCoolRpm_RecFlow9_Y, FFBlw9_X=mTmComprCtrl_n_u16KiCmpCoolRpm_RecFlow9_X}
      mask DialogControl ParameterGroupVar Prompt: 参数
  Flow2Rpm1 : Subsystem  mask{BlwHeatLevel_db=cTmComprCtrl_D_u8HvacFlowTable_db, BlwHeatLevel_sw=cTmComprCtrl_D_u8HvacFlowTable_sw, FFBlw1=mTmComprCtrl_n_u16KiCmpCoolRpm_OsaFlow1, FFBlw1_Y=mTmComprCtrl_n_u16KiCmpCoolRpm_OsaFlow1_Y, FFBlw1_X=mTmComprCtrl_n_u16KiCmpCoolRpm_OsaFlow1_X, FFBlw3=mTmComprCtrl_n_u16KiCmpCoolRpm_OsaFlow3, FFBlw3_Y=mTmComprCtrl_n_u16KiCmpCoolRpm_OsaFlow3_Y, FFBlw3_X=mTmComprCtrl_n_u16KiCmpCoolRpm_OsaFlow3_X, FFBlw5=mTmComprCtrl_n_u16KiCmpCoolRpm_OsaFlow5, FFBlw5_Y=mTmComprCtrl_n_u16KiCmpCoolRpm_OsaFlow5_Y, FFBlw5_X=mTmComprCtrl_n_u16KiCmpCoolRpm_OsaFlow5_X, FFBlw7=mTmComprCtrl_n_u16KiCmpCoolRpm_OsaFlow7, FFBlw7_Y=mTmComprCtrl_n_u16KiCmpCoolRpm_OsaFlow7_Y, FFBlw7_X=mTmComprCtrl_n_u16KiCmpCoolRpm_OsaFlow7_X, FFBlw9=mTmComprCtrl_n_u16KiCmpCoolRpm_OsaFlow9, FFBlw9_Y=mTmComprCtrl_n_u16KiCmpCoolRpm_OsaFlow9_Y, FFBlw9_X=mTmComprCtrl_n_u16KiCmpCoolRpm_OsaFlow9_X}
      mask DialogControl ParameterGroupVar Prompt: 参数
  interpolation : PCMULib/Calculation/interpolation  SystemSampleTime=-1  VariantActivationTime=update diagram  Latency=0  AutoFrameSizeCalculation=off
      settings: SourceProductName=PCMULib
  SM2Ki : Outport
  wires:
  Error/1 -> [Error]
  ? -> [sTmSigProces_Te_s32TAmb]
  sTmIn_X_s32ClimtRcirc/1 -> [sTmIn_X_s32ClimtRcirc]
  sTmComprCtrl_D_u8HvacFlowLevel/1 -> [sTmComprCtrl_D_u8HvacFlowLevel]
  Flow2Rpm/1(Flow2Rpm) -> interpolation/2  "mask"
  [sTmSigProces_Te_s32TAmb] -> Flow2Rpm/2(breakpoint1)
  [Error] -> Flow2Rpm/3(breakpoint2)
  [sTmComprCtrl_D_u8HvacFlowLevel] -> Flow2Rpm1/1(md_u8Blw)
  [sTmSigProces_Te_s32TAmb] -> Flow2Rpm1/2(breakpoint1)
  [sTmIn_X_s32ClimtRcirc] -> interpolation/1
  [sTmComprCtrl_D_u8HvacFlowLevel] -> Flow2Rpm/1(md_u8Blw)
  interpolation/1 -> SM2Ki/1
  Flow2Rpm1/1(Flow2Rpm) -> interpolation/3  "mask"
  [Error] -> Flow2Rpm1/3(breakpoint2)

== system ScriptDemo/Create/createMerge/After/SM3SM23/SM3_Ki/SM3SM1LikeKi ==
  sTmSigProces_D_u8BattThermReq : Inport
  sTmIn_D_u8DCChrgSt : Inport  Port=2
  sTmSigProces_D_u8HvBattCoolgReq : Inport  Port=3
  error : Inport  Port=4
  2-D Lookup Table5 : Lookup_n-D  LookupTableObject=mTmComprCtrl_n_u16FFBattCooltRpmCharging  BreakpointsForDimension1=mTmComprCtrl_n_u16KiSM3BattCooltRpmNorm_Y  BreakpointsForDimension2=mTmComprCtrl_n_u16KiSM3BattCooltRpmNorm_X  BreakpointsForDimension1DataTypeStr=Inherit: Inherit from 'Breakpoint data'  BreakpointsForDimension2DataTypeStr=Inherit: Inherit from 'Breakpoint data'  Table=mTmComprCtrl_n_u16KiSM3BattCooltRpmNorm  TableDataTypeStr=Inherit: Inherit from 'Table data'  ExtrapMethod=Clip  InternalRulePriority=Speed  OutDataTypeStr=Inherit: Inherit via back propagation  RndMeth=Simplest  InputSameDT=off
      settings: InputPortMap=u0,u1
  2-D Lookup Table6 : Lookup_n-D  LookupTableObject=mTmComprCtrl_n_u16FFBattCooltRpmCharging  BreakpointsForDimension1=mTmComprCtrl_n_u16KiSM3BattCooltRpmCharging_Y  BreakpointsForDimension2=mTmComprCtrl_n_u16KiSM3BattCooltRpmCharging_X  BreakpointsForDimension1DataTypeStr=Inherit: Inherit from 'Breakpoint data'  BreakpointsForDimension2DataTypeStr=Inherit: Inherit from 'Breakpoint data'  Table=mTmComprCtrl_n_u16KiSM3BattCooltRpmCharging  TableDataTypeStr=Inherit: Inherit from 'Table data'  ExtrapMethod=Clip  InternalRulePriority=Speed  OutDataTypeStr=Inherit: Inherit via back propagation  RndMeth=Simplest  InputSameDT=off
      settings: InputPortMap=u0,u1
  2-D Lookup Table7 : Lookup_n-D  LookupTableObject=mTmComprCtrl_n_u16FFBattCooltRpmCharging  BreakpointsForDimension1=mTmComprCtrl_n_u16KiSM3BattCooltRpmSuperCharging_Y  BreakpointsForDimension2=mTmComprCtrl_n_u16KiSM3BattCooltRpmSuperCharging_X  BreakpointsForDimension1DataTypeStr=Inherit: Inherit from 'Breakpoint data'  BreakpointsForDimension2DataTypeStr=Inherit: Inherit from 'Breakpoint data'  Table=mTmComprCtrl_n_u16KiSM3BattCooltRpmSuperCharging  TableDataTypeStr=Inherit: Inherit from 'Table data'  ExtrapMethod=Clip  InternalRulePriority=Speed  OutDataTypeStr=Inherit: Inherit via back propagation  RndMeth=Simplest  InputSameDT=off
      settings: InputPortMap=u0,u1
  tableChoose : Subsystem
  Ki : Outport  OutDataTypeStr=uint16
  wires:
  sTmIn_D_u8DCChrgSt/1 -> tableChoose/2(sTmIn_D_u8DCChrgSt)
  sTmSigProces_D_u8BattThermReq/1 -> tableChoose/1(sTmSigProces_D_u8BattThermReq)
  2-D Lookup Table7/1 -> tableChoose/5(tab3)
  2-D Lookup Table5/1 -> tableChoose/3(tab1)
  2-D Lookup Table6/1 -> tableChoose/4(tab2)
  sTmSigProces_D_u8HvBattCoolgReq/1 -> 2-D Lookup Table7/1, 2-D Lookup Table6/1, 2-D Lookup Table5/1
  error/1 -> 2-D Lookup Table7/2, 2-D Lookup Table6/2, 2-D Lookup Table5/2
  tableChoose/1(out) -> Ki/1

== system ScriptDemo/Create/createMerge/After/SM3SM23/SM3_Ki/SM3SM2LikeKi ==
  Error : Inport
  sTmIn_X_s32ClimtRcirc : Inport  Port=2  OutDataTypeStr=single
  sTmComprCtrl_D_u8HvacFlowLevel : Inport  Port=3  OutDataTypeStr=uint8
  Osa : Subsystem  mask{BlwHeatLevel_db=cTmComprCtrl_D_u8HvacFlowTable_db, BlwHeatLevel_sw=cTmComprCtrl_D_u8HvacFlowTable_sw, FFBlw1=mTmComprCtrl_n_u16KiSM3CmpCoolRpm_OsaFlow1, FFBlw1_Y=mTmComprCtrl_n_u16KiSM3CmpCoolRpm_OsaFlow1_Y, FFBlw1_X=mTmComprCtrl_n_u16KiSM3CmpCoolRpm_OsaFlow1_X, FFBlw3=mTmComprCtrl_n_u16KiSM3CmpCoolRpm_OsaFlow3, FFBlw3_Y=mTmComprCtrl_n_u16KiSM3CmpCoolRpm_OsaFlow3_Y, FFBlw3_X=mTmComprCtrl_n_u16KiSM3CmpCoolRpm_OsaFlow3_X, FFBlw5=mTmComprCtrl_n_u16KiSM3CmpCoolRpm_OsaFlow5, FFBlw5_Y=mTmComprCtrl_n_u16KiSM3CmpCoolRpm_OsaFlow5_Y, FFBlw5_X=mTmComprCtrl_n_u16KiSM3CmpCoolRpm_OsaFlow5_X, FFBlw7=mTmComprCtrl_n_u16KiSM3CmpCoolRpm_OsaFlow7, FFBlw7_Y=mTmComprCtrl_n_u16KiSM3CmpCoolRpm_OsaFlow7_Y, FFBlw7_X=mTmComprCtrl_n_u16KiSM3CmpCoolRpm_OsaFlow7_X, FFBlw9=mTmComprCtrl_n_u16KiSM3CmpCoolRpm_OsaFlow9, FFBlw9_Y=mTmComprCtrl_n_u16KiSM3CmpCoolRpm_OsaFlow9_Y, FFBlw9_X=mTmComprCtrl_n_u16KiSM3CmpCoolRpm_OsaFlow9_X}
      mask DialogControl ParameterGroupVar Prompt: 参数
  Rec : Subsystem  mask{BlwHeatLevel_db=cTmComprCtrl_D_u8HvacFlowTable_db, BlwHeatLevel_sw=cTmComprCtrl_D_u8HvacFlowTable_sw, FFBlw1=mTmComprCtrl_n_u16KiSM3CmpCoolRpm_RecFlow1, FFBlw1_Y=mTmComprCtrl_n_u16KiSM3CmpCoolRpm_RecFlow1_Y, FFBlw1_X=mTmComprCtrl_n_u16KiSM3CmpCoolRpm_RecFlow1_X, FFBlw3=mTmComprCtrl_n_u16KiSM3CmpCoolRpm_RecFlow3, FFBlw3_Y=mTmComprCtrl_n_u16KiSM3CmpCoolRpm_RecFlow3_Y, FFBlw3_X=mTmComprCtrl_n_u16KiSM3CmpCoolRpm_RecFlow3_X, FFBlw5=mTmComprCtrl_n_u16KiSM3CmpCoolRpm_RecFlow5, FFBlw5_Y=mTmComprCtrl_n_u16KiSM3CmpCoolRpm_RecFlow5_Y, FFBlw5_X=mTmComprCtrl_n_u16KiSM3CmpCoolRpm_RecFlow5_X, FFBlw7=mTmComprCtrl_n_u16KiSM3CmpCoolRpm_RecFlow7, FFBlw7_Y=mTmComprCtrl_n_u16KiSM3CmpCoolRpm_RecFlow7_Y, FFBlw7_X=mTmComprCtrl_n_u16KiSM3CmpCoolRpm_RecFlow7_X, FFBlw9=mTmComprCtrl_n_u16KiSM3CmpCoolRpm_RecFlow9, FFBlw9_Y=mTmComprCtrl_n_u16KiSM3CmpCoolRpm_RecFlow9_Y, FFBlw9_X=mTmComprCtrl_n_u16KiSM3CmpCoolRpm_RecFlow9_X}
      mask DialogControl ParameterGroupVar Prompt: 参数
  interpolation : PCMULib/Calculation/interpolation  SystemSampleTime=-1  VariantActivationTime=update diagram  Latency=0  AutoFrameSizeCalculation=off
      settings: SourceProductName=PCMULib
  Ki : Outport
  wires:
  interpolation/1 -> Ki/1
  [sTmIn_X_s32ClimtRcirc] -> interpolation/1
  Error/1 -> [Error]
  ? -> [sTmSigProces_Te_s32TAmb]
  sTmIn_X_s32ClimtRcirc/1 -> [sTmIn_X_s32ClimtRcirc]
  sTmComprCtrl_D_u8HvacFlowLevel/1 -> [sTmComprCtrl_D_u8HvacFlowLevel]
  [sTmComprCtrl_D_u8HvacFlowLevel] -> Rec/1(md_u8Blw)
  [sTmSigProces_Te_s32TAmb] -> Rec/2(breakpoint1)
  [Error] -> Rec/3(breakpoint2)
  [sTmComprCtrl_D_u8HvacFlowLevel] -> Osa/1(md_u8Blw)
  [sTmSigProces_Te_s32TAmb] -> Osa/2(breakpoint1)
  [Error] -> Osa/3(breakpoint2)
  Rec/1(Flow2Rpm) -> interpolation/2  "mask"
  Osa/1(Flow2Rpm) -> interpolation/3  "mask"

== system ScriptDemo/Create/createMerge/After/SM3SM23/SM3_Kp/SM1Kp ==
  sTmSigProces_D_u8BattThermReq : Inport
  sTmIn_D_u8DCChrgSt : Inport  Port=2
  sTmSigProces_D_u8HvBattCoolgReq : Inport  Port=3
  Error : Inport  Port=4
  2-D Lookup Table5 : Lookup_n-D  LookupTableObject=mTmComprCtrl_n_u16FFBattCooltRpmCharging  BreakpointsForDimension1=mTmComprCtrl_n_u16KpBattCooltRpmNorm_Y  BreakpointsForDimension2=mTmComprCtrl_n_u16KpBattCooltRpmNorm_X  BreakpointsForDimension1DataTypeStr=Inherit: Inherit from 'Breakpoint data'  BreakpointsForDimension2DataTypeStr=Inherit: Inherit from 'Breakpoint data'  Table=mTmComprCtrl_n_u16KpBattCooltRpmNorm  TableDataTypeStr=Inherit: Inherit from 'Table data'  ExtrapMethod=Clip  InternalRulePriority=Speed  OutDataTypeStr=Inherit: Inherit via back propagation  RndMeth=Simplest  InputSameDT=off
      settings: InputPortMap=u0,u1
  2-D Lookup Table6 : Lookup_n-D  LookupTableObject=mTmComprCtrl_n_u16FFBattCooltRpmCharging  BreakpointsForDimension1=mTmComprCtrl_n_u16KpBattCooltRpmCharging_Y  BreakpointsForDimension2=mTmComprCtrl_n_u16KpBattCooltRpmCharging_X  BreakpointsForDimension1DataTypeStr=Inherit: Inherit from 'Breakpoint data'  BreakpointsForDimension2DataTypeStr=Inherit: Inherit from 'Breakpoint data'  Table=mTmComprCtrl_n_u16KpBattCooltRpmCharging  TableDataTypeStr=Inherit: Inherit from 'Table data'  ExtrapMethod=Clip  InternalRulePriority=Speed  OutDataTypeStr=Inherit: Inherit via back propagation  RndMeth=Simplest  InputSameDT=off
      settings: InputPortMap=u0,u1
  2-D Lookup Table7 : Lookup_n-D  LookupTableObject=mTmComprCtrl_n_u16FFBattCooltRpmCharging  BreakpointsForDimension1=mTmComprCtrl_n_u16KpBattCooltRpmSuperCharging_Y  BreakpointsForDimension2=mTmComprCtrl_n_u16KpBattCooltRpmSuperCharging_X  BreakpointsForDimension1DataTypeStr=Inherit: Inherit from 'Breakpoint data'  BreakpointsForDimension2DataTypeStr=Inherit: Inherit from 'Breakpoint data'  Table=mTmComprCtrl_n_u16KpBattCooltRpmSuperCharging  TableDataTypeStr=Inherit: Inherit from 'Table data'  ExtrapMethod=Clip  InternalRulePriority=Speed  OutDataTypeStr=Inherit: Inherit via back propagation  RndMeth=Simplest  InputSameDT=off
      settings: InputPortMap=u0,u1
  tableChoose : Subsystem
  SM1Kp : Outport
  wires:
  sTmIn_D_u8DCChrgSt/1 -> tableChoose/2(sTmIn_D_u8DCChrgSt)
  sTmSigProces_D_u8BattThermReq/1 -> tableChoose/1(sTmSigProces_D_u8BattThermReq)
  2-D Lookup Table7/1 -> tableChoose/5(tab3)
  2-D Lookup Table5/1 -> tableChoose/3(tab1)
  2-D Lookup Table6/1 -> tableChoose/4(tab2)
  tableChoose/1(out) -> SM1Kp/1
  sTmSigProces_D_u8HvBattCoolgReq/1 -> 2-D Lookup Table7/1, 2-D Lookup Table6/1, 2-D Lookup Table5/1
  Error/1 -> 2-D Lookup Table7/2, 2-D Lookup Table6/2, 2-D Lookup Table5/2

== system ScriptDemo/Create/createMerge/After/SM3SM23/SM3_Kp/SM2Kp ==
  Error : Inport
  sTmIn_X_s32ClimtRcirc : Inport  Port=2  OutDataTypeStr=single
  sTmComprCtrl_D_u8HvacFlowLevel : Inport  Port=3  OutDataTypeStr=uint8
  Osa : Subsystem  mask{BlwHeatLevel_db=cTmComprCtrl_D_u8HvacFlowTable_db, BlwHeatLevel_sw=cTmComprCtrl_D_u8HvacFlowTable_sw, FFBlw1=mTmComprCtrl_n_u16KpCmpCoolRpm_OsaFlow1, FFBlw1_Y=mTmComprCtrl_n_u16KpCmpCoolRpm_OsaFlow1_Y, FFBlw1_X=mTmComprCtrl_n_u16KpCmpCoolRpm_OsaFlow1_X, FFBlw3=mTmComprCtrl_n_u16KpCmpCoolRpm_OsaFlow3, FFBlw3_Y=mTmComprCtrl_n_u16KpCmpCoolRpm_OsaFlow3_Y, FFBlw3_X=mTmComprCtrl_n_u16KpCmpCoolRpm_OsaFlow3_X, FFBlw5=mTmComprCtrl_n_u16KpCmpCoolRpm_OsaFlow5, FFBlw5_Y=mTmComprCtrl_n_u16KpCmpCoolRpm_OsaFlow5_Y, FFBlw5_X=mTmComprCtrl_n_u16KpCmpCoolRpm_OsaFlow5_X, FFBlw7=mTmComprCtrl_n_u16KpCmpCoolRpm_OsaFlow7, FFBlw7_Y=mTmComprCtrl_n_u16KpCmpCoolRpm_OsaFlow7_Y, FFBlw7_X=mTmComprCtrl_n_u16KpCmpCoolRpm_OsaFlow7_X, FFBlw9=mTmComprCtrl_n_u16KpCmpCoolRpm_OsaFlow9, FFBlw9_Y=mTmComprCtrl_n_u16KpCmpCoolRpm_OsaFlow9_Y, FFBlw9_X=mTmComprCtrl_n_u16KpCmpCoolRpm_OsaFlow9_X}
      mask DialogControl ParameterGroupVar Prompt: 参数
  Rec : Subsystem  mask{BlwHeatLevel_db=cTmComprCtrl_D_u8HvacFlowTable_db, BlwHeatLevel_sw=cTmComprCtrl_D_u8HvacFlowTable_sw, FFBlw1=mTmComprCtrl_n_u16KpCmpCoolRpm_RecFlow1, FFBlw1_Y=mTmComprCtrl_n_u16KpCmpCoolRpm_RecFlow1_Y, FFBlw1_X=mTmComprCtrl_n_u16KpCmpCoolRpm_RecFlow1_X, FFBlw3=mTmComprCtrl_n_u16KpCmpCoolRpm_RecFlow3, FFBlw3_Y=mTmComprCtrl_n_u16KpCmpCoolRpm_RecFlow3_Y, FFBlw3_X=mTmComprCtrl_n_u16KpCmpCoolRpm_RecFlow3_X, FFBlw5=mTmComprCtrl_n_u16KpCmpCoolRpm_RecFlow5, FFBlw5_Y=mTmComprCtrl_n_u16KpCmpCoolRpm_RecFlow5_Y, FFBlw5_X=mTmComprCtrl_n_u16KpCmpCoolRpm_RecFlow5_X, FFBlw7=mTmComprCtrl_n_u16KpCmpCoolRpm_RecFlow7, FFBlw7_Y=mTmComprCtrl_n_u16KpCmpCoolRpm_RecFlow7_Y, FFBlw7_X=mTmComprCtrl_n_u16KpCmpCoolRpm_RecFlow7_X, FFBlw9=mTmComprCtrl_n_u16KpCmpCoolRpm_RecFlow9, FFBlw9_Y=mTmComprCtrl_n_u16KpCmpCoolRpm_RecFlow9_Y, FFBlw9_X=mTmComprCtrl_n_u16KpCmpCoolRpm_RecFlow9_X}
      mask DialogControl ParameterGroupVar Prompt: 参数
  interpolation : PCMULib/Calculation/interpolation  SystemSampleTime=-1  VariantActivationTime=update diagram  Latency=0  AutoFrameSizeCalculation=off
      settings: SourceProductName=PCMULib
  SM2Kp : Outport
  wires:
  Error/1 -> [Error]
  ? -> [sTmSigProces_Te_s32TAmb]
  sTmIn_X_s32ClimtRcirc/1 -> [sTmIn_X_s32ClimtRcirc]
  sTmComprCtrl_D_u8HvacFlowLevel/1 -> [sTmComprCtrl_D_u8HvacFlowLevel]
  [Error] -> Rec/3(breakpoint2)
  [sTmSigProces_Te_s32TAmb] -> Rec/2(breakpoint1)
  Osa/1(Flow2Rpm) -> interpolation/3  "mask"
  [sTmIn_X_s32ClimtRcirc] -> interpolation/1
  [sTmComprCtrl_D_u8HvacFlowLevel] -> Rec/1(md_u8Blw)
  [Error] -> Osa/3(breakpoint2)
  [sTmSigProces_Te_s32TAmb] -> Osa/2(breakpoint1)
  Rec/1(Flow2Rpm) -> interpolation/2  "mask"
  [sTmComprCtrl_D_u8HvacFlowLevel] -> Osa/1(md_u8Blw)
  interpolation/1 -> SM2Kp/1

== system ScriptDemo/Create/createMerge/After/SM3SM23/SM3_Kp/SM3SM1LikeKp ==
  sTmSigProces_D_u8BattThermReq : Inport
  sTmIn_D_u8DCChrgSt : Inport  Port=2
  sTmSigProces_D_u8HvBattCoolgReq : Inport  Port=3
  error : Inport  Port=4
  2-D Lookup Table5 : Lookup_n-D  LookupTableObject=mTmComprCtrl_n_u16FFBattCooltRpmCharging  BreakpointsForDimension1=mTmComprCtrl_n_u16KpSM3BattCooltRpmNorm_Y  BreakpointsForDimension2=mTmComprCtrl_n_u16KpSM3BattCooltRpmNorm_X  BreakpointsForDimension1DataTypeStr=Inherit: Inherit from 'Breakpoint data'  BreakpointsForDimension2DataTypeStr=Inherit: Inherit from 'Breakpoint data'  Table=mTmComprCtrl_n_u16KpSM3BattCooltRpmNorm  TableDataTypeStr=Inherit: Inherit from 'Table data'  ExtrapMethod=Clip  InternalRulePriority=Speed  OutDataTypeStr=Inherit: Inherit via back propagation  RndMeth=Simplest  InputSameDT=off
      settings: InputPortMap=u0,u1
  2-D Lookup Table6 : Lookup_n-D  LookupTableObject=mTmComprCtrl_n_u16FFBattCooltRpmCharging  BreakpointsForDimension1=mTmComprCtrl_n_u16KpSM3BattCooltRpmCharging_Y  BreakpointsForDimension2=mTmComprCtrl_n_u16KpSM3BattCooltRpmCharging_X  BreakpointsForDimension1DataTypeStr=Inherit: Inherit from 'Breakpoint data'  BreakpointsForDimension2DataTypeStr=Inherit: Inherit from 'Breakpoint data'  Table=mTmComprCtrl_n_u16KpSM3BattCooltRpmCharging  TableDataTypeStr=Inherit: Inherit from 'Table data'  ExtrapMethod=Clip  InternalRulePriority=Speed  OutDataTypeStr=Inherit: Inherit via back propagation  RndMeth=Simplest  InputSameDT=off
      settings: InputPortMap=u0,u1
  2-D Lookup Table7 : Lookup_n-D  LookupTableObject=mTmComprCtrl_n_u16FFBattCooltRpmCharging  BreakpointsForDimension1=mTmComprCtrl_n_u16KpSM3BattCooltRpmSuperCharging_Y  BreakpointsForDimension2=mTmComprCtrl_n_u16KpSM3BattCooltRpmSuperCharging_X  BreakpointsForDimension1DataTypeStr=Inherit: Inherit from 'Breakpoint data'  BreakpointsForDimension2DataTypeStr=Inherit: Inherit from 'Breakpoint data'  Table=mTmComprCtrl_n_u16KpSM3BattCooltRpmSuperCharging  TableDataTypeStr=Inherit: Inherit from 'Table data'  ExtrapMethod=Clip  InternalRulePriority=Speed  OutDataTypeStr=Inherit: Inherit via back propagation  RndMeth=Simplest  InputSameDT=off
      settings: InputPortMap=u0,u1
  tableChoose : Subsystem
  Kp : Outport
  wires:
  sTmIn_D_u8DCChrgSt/1 -> tableChoose/2(sTmIn_D_u8DCChrgSt)
  sTmSigProces_D_u8BattThermReq/1 -> tableChoose/1(sTmSigProces_D_u8BattThermReq)
  2-D Lookup Table7/1 -> tableChoose/5(tab3)
  2-D Lookup Table5/1 -> tableChoose/3(tab1)
  2-D Lookup Table6/1 -> tableChoose/4(tab2)
  sTmSigProces_D_u8HvBattCoolgReq/1 -> 2-D Lookup Table7/1, 2-D Lookup Table6/1, 2-D Lookup Table5/1
  error/1 -> 2-D Lookup Table7/2, 2-D Lookup Table6/2, 2-D Lookup Table5/2
  tableChoose/1(out) -> Kp/1
